simulink model "bh_2dof_NP_CONTROLLED"  (R2017a)
settings: Solver=ode45  StartTime=0.0  StopTime=70  FixedStep=0.001  RelTol=1e-7  EnableMultiTasking=on
values from neighbouring files (symbols this model uses):
  theta1_0 = 0    [bh_SIMPARAMS_for_2dof_NP_Control_sim.m]
  theta1_dot_0 = 0    [bh_SIMPARAMS_for_2dof_NP_Control_sim.m]
  theta4_0 = 0    [bh_SIMPARAMS_for_2dof_NP_Control_sim.m]
  theta4_dot_0 = 0    [bh_SIMPARAMS_for_2dof_NP_Control_sim.m]
undefined symbols (not defined in the file or in its folder): b1_damp, b4_damp, g, L1x, L1y, L1z, mass1, mass4, Rturn, sigbuilder_block
libraries: simulink_extras x18, simulink x4, discretizing x1
settings Model: Creator=bhorton  LastModifiedBy=bhorton
settings SolverCC: ZeroCrossAlgorithm=Adaptive
settings OptimizationCC: LifeSpan=inf
settings DebuggingCC: SFUnexpectedBacktrackingDiag=warning  SFNoUnconditionalDefaultTransitionDiag=warning  SFExecutionAtInitializationDiag=none
settings GRTTargetCC: TargetLangStandard=C89/C90 (ANSI)
settings ConfigComp: CovMetricSettings=dw  CovHtmlReporting=on  CovSaveCumulativeToWorkspaceVar=on  CovSaveSingleToWorkspaceVar=on  CovExternalEMLEnable=off
settings SimscapeCC: SimscapeLogDataHistory=10000  SelectedTab=Simscape Multibody
settings ExplorerConfigSet: InternalSimMechanicsExplorerSettings="<ExplorerConfiguration><canonicalview>default</canonicalview><AnimationSetting><BasePlaybackSpeed>2</BasePlaybackSpeed><PlaybackSpeedFactor>1.0</PlaybackSpeedFactor></AnimationSetting><TilePanel><TileInfo><Tiles Columns=\"1\" Count=\"1\" Rows=\"1\"><Column Left=\"2\" Weight=\"1\"/><Column Left=\"820\"/><Row Top=\"2\" Weight=\"1\"/><Row Top=\"545\"/><Tile Height=\"1\" Width=\"1\" X=\"0\" Y=\"0\"/></Tiles></TileInfo><SceneInfo><SceneViewer><BGColor><R>0.60000002384185791</R><G>0.60000002384185791</G><B>0.60000002384185791</B></BGColor><Camera><DoPerspective>off</DoPerspective><Position><X>0.3018347345439823</X><Y>0.024415264242792611</Y><Z>0.21433472519445274</Z></Position><Center><X>0.024999999062628675</X><Y>0.30124999972414623</Y><Z>-0.062500010286905439</Z></Center><Up><X>-0.40824829046386751</X><Y>0.40824829046386751</Y><Z>0.81649658092772159</Z></Up><ViewLimDist>1</ViewLimDist><YLim>0.27384785473346712</YLim><XLim>0.4148743716842227</XLim></Camera></SceneViewer></SceneInfo></TilePanel><MechEditorPanel><Cameras/><GfxPanelCameraMap/></MechEditorPanel></ExplorerConfiguration>"

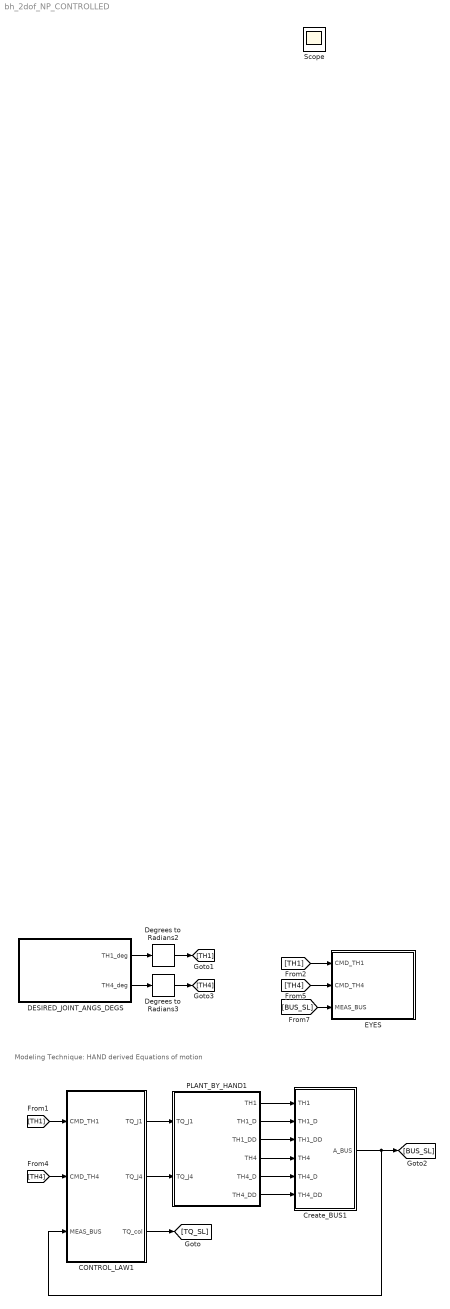
== system bh_2dof_NP_CONTROLLED ==
  note: Modeling Technique: HAND derived Equations of motion
  CONTROL_LAW1 : Subsystem
  Create_BUS1 : Subsystem
  DESIRED_JOINT_ANGS_DEGS : Subsystem  Tag=STV Subsys  LoadFcn=sigbuilder_block('load');  StartFcn=sigbuilder_block('start');  StopFcn=sigbuilder_block('stop');  ClipboardFcn=sigbuilder_block('clipboard');  mask(Sigbuilder block){tuvar=[0:10]}
      mask help: Simulink:masks:SigbuilderBlock_MD
      mask init:
      | if ~strcmp(get_param(bdroot(gcbh),'SimulationStatus'),'stopped') tuvar = sigbuilder_block('maskInit'); end
      settings: CopyFcn=sigbuilder_block('copy');  DeleteFcn=sigbuilder_block('delete');  ModelCloseFcn=sigbuilder_block('modelClose');  PreSaveFcn=sigbuilder_block('preSave');  PauseFcn=sigbuilder_block('pause');  ContinueFcn=sigbuilder_block('continue');  NameChangeFcn=sigbuilder_block('namechange');  OpenFcn=sigbuilder_block('open',[6 30 1428 681.75 ]);  CloseFcn=sigbuilder_block('close');
      mask Display: plot(0, 0, 100, 100,[2, 2, 32, 32, 2], [68, 8, 8, 68, 68],[32, 2], [38, 38], [32, 19, 2],[53, 60, 44], [32, 17, 17, 2],[16, 16, 31, 31]);txt = getActiveGroup(gcbh);text(2, 100, txt,'verticalAlignment', 'top');
  Degrees to Radians2 : simulink_extras/Transformations/Degrees to Radians
  Degrees to Radians3 : simulink_extras/Transformations/Degrees to Radians
  EYES : Subsystem
  PLANT_BY_HAND1 : Subsystem
  Scope : Scope
  wires:
  [TH1] -> EYES/1(CMD_TH1)
  [TH4] -> EYES/2(CMD_TH4)
  [TH1] -> CONTROL_LAW1/1(CMD_TH1)
  CONTROL_LAW1/3(TQ_col) -> [TQ_SL]
  PLANT_BY_HAND1/5(TH4_D) -> Create_BUS1/5(TH4_D)
  [TH4] -> CONTROL_LAW1/2(CMD_TH4)
  PLANT_BY_HAND1/3(TH1_DD) -> Create_BUS1/3(TH1_DD)
  PLANT_BY_HAND1/4(TH4) -> Create_BUS1/4(TH4)
  PLANT_BY_HAND1/1(TH1) -> Create_BUS1/1(TH1)
  PLANT_BY_HAND1/6(TH4_DD) -> Create_BUS1/6(TH4_DD)
  Create_BUS1/1(A_BUS) -> [BUS_SL], CONTROL_LAW1/3(MEAS_BUS)
  PLANT_BY_HAND1/2(TH1_D) -> Create_BUS1/2(TH1_D)
  CONTROL_LAW1/1(TQ_J1) -> PLANT_BY_HAND1/1("TQ_J1 ")
  CONTROL_LAW1/2(TQ_J4) -> PLANT_BY_HAND1/2(TQ_J4)
  [BUS_SL] -> EYES/3(MEAS_BUS)
  Degrees to Radians3/1 -> [TH4]
  DESIRED_JOINT_ANGS_DEGS/1(TH1_deg) -> Degrees to Radians2/1
  Degrees to Radians2/1 -> [TH1]
  DESIRED_JOINT_ANGS_DEGS/2(TH4_deg) -> Degrees to Radians3/1

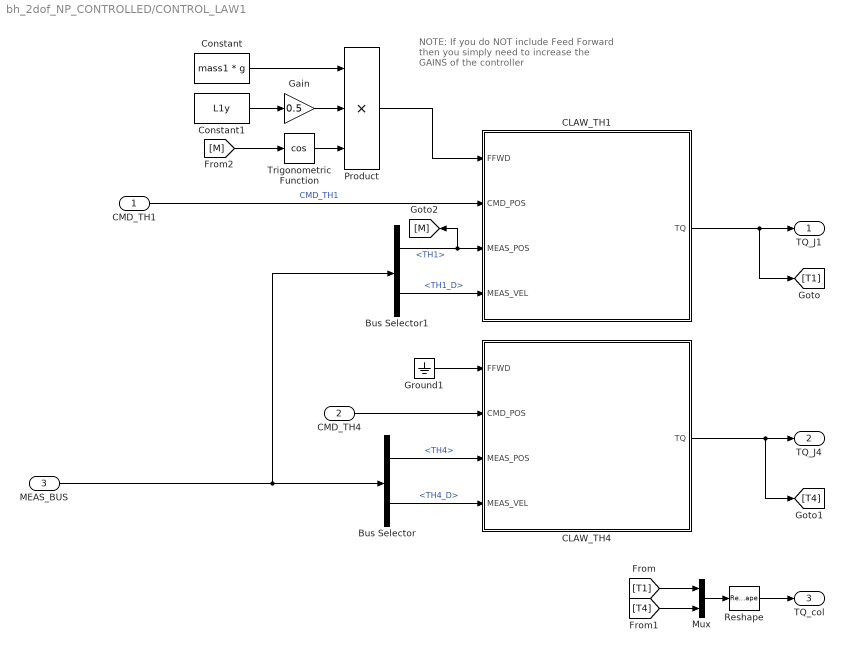
== system bh_2dof_NP_CONTROLLED/CONTROL_LAW1 ==
  note: NOTE:
      | If you do NOT include Feed Forward
      | then you simply need to increase the GAINS of the controller
  CMD_TH1 : Inport
  CMD_TH4 : Inport  Port=2
  MEAS_BUS : Inport  Port=3
  Bus Selector : BusSelector  OutputSignals=TH4,TH4_D
  Bus Selector1 : BusSelector  OutputSignals=TH1,TH1_D
  CLAW_TH1 : Subsystem
  CLAW_TH4 : Subsystem
  Constant : Constant  Value=mass1 * g
  Constant1 : Constant  Value=L1y
  Gain : Gain  Gain=0.5
  Ground1 : Ground
  Mux : Mux  Inputs=2
  Product : Product  Inputs=3
  Reshape : Reshape  OutputDimensionality=Column vector (2-D)
  Trigonometric Function : Trigonometry  Operator=cos
  TQ_J1 : Outport
  TQ_J4 : Outport  Port=2
  TQ_col : Outport  Port=3
  wires:
  MEAS_BUS/1 -> Bus Selector1/1, Bus Selector/1
  CMD_TH4/1 -> CLAW_TH4/2(CMD_POS)
  Bus Selector/2 -> CLAW_TH4/4(MEAS_VEL)  "<TH4_D>"
  Bus Selector/1 -> CLAW_TH4/3(MEAS_POS)  "<TH4>"
  Bus Selector1/1 -> [M], CLAW_TH1/3(MEAS_POS)  "<TH1>"
  Bus Selector1/2 -> CLAW_TH1/4(MEAS_VEL)  "<TH1_D>"
  CLAW_TH1/1(TQ) -> [T1], TQ_J1/1
  Ground1/1 -> CLAW_TH4/1(FFWD)
  CLAW_TH4/1(TQ) -> [T4], TQ_J4/1
  CMD_TH1/1 -> CLAW_TH1/2(CMD_POS)  "CMD_TH1"
  Constant/1 -> Product/1
  Constant1/1 -> Gain/1
  Product/1 -> CLAW_TH1/1(FFWD)
  Gain/1 -> Product/2
  Trigonometric Function/1 -> Product/3
  Mux/1 -> Reshape/1
  [T1] -> Mux/1
  [T4] -> Mux/2
  Reshape/1 -> TQ_col/1
  [M] -> Trigonometric Function/1

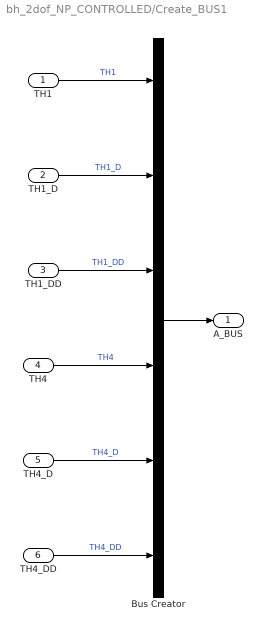
== system bh_2dof_NP_CONTROLLED/Create_BUS1 ==
  TH1 : Inport
  TH1_D : Inport  Port=2
  TH1_DD : Inport  Port=3
  TH4 : Inport  Port=4
  TH4_D : Inport  Port=5
  TH4_DD : Inport  Port=6
  Bus Creator : BusCreator  Inputs=6
  A_BUS : Outport
  wires:
  TH1_DD/1 -> Bus Creator/3  "TH1_DD"
  TH1_D/1 -> Bus Creator/2  "TH1_D"
  TH1/1 -> Bus Creator/1  "TH1"
  Bus Creator/1 -> A_BUS/1
  TH4_DD/1 -> Bus Creator/6  "TH4_DD"
  TH4_D/1 -> Bus Creator/5  "TH4_D"
  TH4/1 -> Bus Creator/4  "TH4"

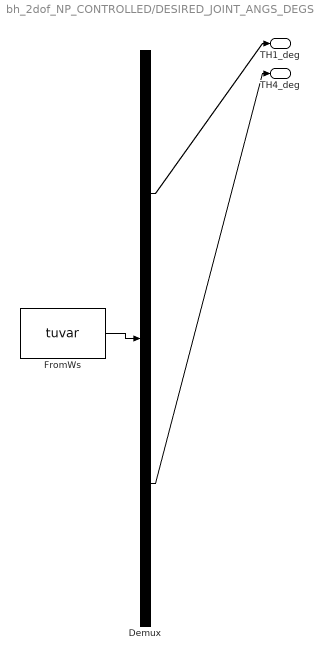
== system bh_2dof_NP_CONTROLLED/DESIRED_JOINT_ANGS_DEGS ==
  Demux : Demux  Tag=STV Demux  Outputs=2
  FromWs : FromWorkspace  Tag=STV FromWs  VariableName=tuvar  SampleTime=0
      SigBuilderData=|
      | common.afterFinalStr = 'Extrapolate'
      | common.sampleTime = 0
      | dataSet(1).timeRange = [0 60]
      | dataSet(1).name = 'SCENARIO_A_JUST_TH1'
      | dataSet(2).timeRange = [0 60]
      | dataSet(2).name = 'SCENARIO_B_JUST_TH4'
      | dataSet(3).timeRange = [0 60]
      | dataSet(3).name = 'SCENARIO_C_TH1_and_TH4'
      | dataSet(4).timeRange = [0 60]
      | dataSet(4).name = 'SCENARIO_D_TH1_and_TH4'
      | dataSet(5).timeRange = [0 70]
      | dataSet(5).name = 'SCENARIO_E'
      | sbobj.Groups(1).Name = 'SCENARIO_A_JUST_TH1'
      | sbobj.Groups(1).Signals(1).Name = 'TH1_deg'
      | sbobj.Groups(1).Signals(1).XData = [0 20 20 60]
      | sbobj.Groups(1).Signals(1).YData = [0 0 45 45]
      | sbobj.Groups(1).Signals(2).Name = 'TH4_deg'
      | sbobj.Groups(1).Signals(2).XData = [0 60]
      | sbobj.Groups(1).Signals(2).YData = [0 0]
      | sbobj.Groups(1).TimeRange = [0 60]
      | sbobj.Groups(2).Name = 'SCENARIO_B_JUST_TH4'
      | sbobj.Groups(2).Signals(1).Name = 'TH1_deg'
      | sbobj.Groups(2).Signals(1).XData = [0 20 60]
      | sbobj.Groups(2).Signals(1).YData = [0 0 0]
      | sbobj.Groups(2).Signals(2).Name = 'TH4_deg'
      | sbobj.Groups(2).Signals(2).XData = [0 20 20 60]
      | sbobj.Groups(2).Signals(2).YData = [0 0 45 45]
      | sbobj.Groups(2).TimeRange = [0 60]
      | sbobj.Groups(3).Name = 'SCENARIO_C_TH1_and_TH4'
      | sbobj.Groups(3).Signals(1).Name = 'TH1_deg'
      | sbobj.Groups(3).Signals(1).XData = [0 10 10 40 60]
      | sbobj.Groups(3).Signals(1).YData = [0 0 45 45 0]
      | sbobj.Groups(3).Signals(2).Name = 'TH4_deg'
      | sbobj.Groups(3).Signals(2).XData = [0 14.95 14.95 30 60]
      | sbobj.Groups(3).Signals(2).YData = [0 0 45 45 0]
      | sbobj.Groups(3).TimeRange = [0 60]
      | sbobj.Groups(4).Name = 'SCENARIO_D_TH1_and_TH4'
      | sbobj.Groups(4).Signals(1).Name = 'TH1_deg'
      | sbobj.Groups(4).Signals(1).XData = [0 10 40 60]
      | sbobj.Groups(4).Signals(1).YData = [0 45 45 0]
      | sbobj.Groups(4).Signals(2).Name = 'TH4_deg'
      | sbobj.Groups(4).Signals(2).XData = [0 10 30 60]
      | sbobj.Groups(4).Signals(2).YData = [0 45 45 0]
      | sbobj.Groups(4).TimeRange = [0 60]
      | sbobj.Groups(5).Name = 'SCENARIO_E'
      | sbobj.Groups(5).Signals(1).Name = 'TH1_deg'
      | sbobj.Groups(5).Signals(1).XData = [0 35.15 45.4 60 70]
      | sbobj.Groups(5).Signals(1).YData = [0 0 45 -45 0]
      | sbobj.Groups(5).Signals(2).Name = 'TH4_deg'
      | sbobj.Groups(5).Signals(2).XData = [0 10 25 30 70]
      | sbobj.Groups(5).Signals(2).YData = [0 -90 90 0 0]
      | sbobj.Groups(5).TimeRange = [0 70]
  TH1_deg : Outport  Tag=STV Outport
  TH4_deg : Outport  Tag=STV Outport  Port=2
  wires:
  FromWs/1 -> Demux/1
  Demux/1 -> TH1_deg/1
  Demux/2 -> TH4_deg/1

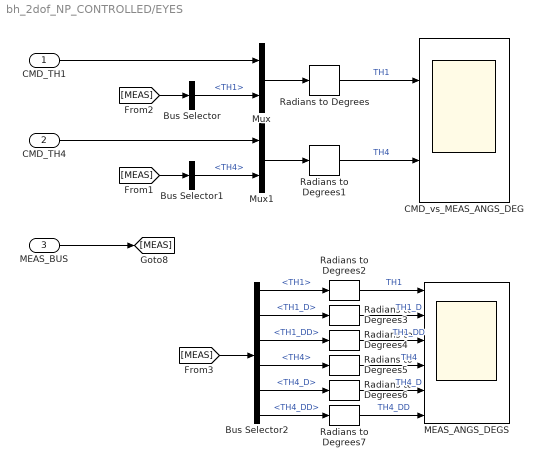
== system bh_2dof_NP_CONTROLLED/EYES ==
  CMD_TH1 : Inport
  CMD_TH4 : Inport  Port=2
  MEAS_BUS : Inport  Port=3
  Bus Selector : BusSelector  OutputSignals=TH1
  Bus Selector1 : BusSelector  OutputSignals=TH4
  Bus Selector2 : BusSelector  OutputSignals=TH1,TH1_D,TH1_DD,TH4,TH4_D,TH4_DD
  CMD_vs_MEAS_ANGS_DEG : Scope  NumInputPorts=2
  MEAS_ANGS_DEGS : Scope  NumInputPorts=6
  Mux : Mux  Inputs=2
  Mux1 : Mux  Inputs=2
  Radians to Degrees{,1..7} (8 alike) : simulink_extras/Transformations/Radians to Degrees
  wires:
  MEAS_BUS/1 -> [MEAS]
  CMD_TH1/1 -> Mux/1
  Bus Selector/1 -> Mux/2  "<TH1>"
  [MEAS] -> Bus Selector/1
  Mux/1 -> Radians to Degrees/1
  CMD_TH4/1 -> Mux1/1
  Bus Selector1/1 -> Mux1/2  "<TH4>"
  [MEAS] -> Bus Selector1/1
  Mux1/1 -> Radians to Degrees1/1
  Radians to Degrees1/1 -> CMD_vs_MEAS_ANGS_DEG/2  "TH4"
  Radians to Degrees/1 -> CMD_vs_MEAS_ANGS_DEG/1  "TH1"
  [MEAS] -> Bus Selector2/1
  Bus Selector2/6 -> Radians to Degrees7/1  "<TH4_DD>"
  Bus Selector2/3 -> Radians to Degrees4/1  "<TH1_DD>"
  Bus Selector2/4 -> Radians to Degrees5/1  "<TH4>"
  Bus Selector2/5 -> Radians to Degrees6/1  "<TH4_D>"
  Bus Selector2/2 -> Radians to Degrees3/1  "<TH1_D>"
  Bus Selector2/1 -> Radians to Degrees2/1  "<TH1>"
  Radians to Degrees2/1 -> MEAS_ANGS_DEGS/1  "TH1"
  Radians to Degrees3/1 -> MEAS_ANGS_DEGS/2  "TH1_D"
  Radians to Degrees4/1 -> MEAS_ANGS_DEGS/3  "TH1_DD"
  Radians to Degrees5/1 -> MEAS_ANGS_DEGS/4  "TH4"
  Radians to Degrees6/1 -> MEAS_ANGS_DEGS/5  "TH4_D"
  Radians to Degrees7/1 -> MEAS_ANGS_DEGS/6  "TH4_DD"

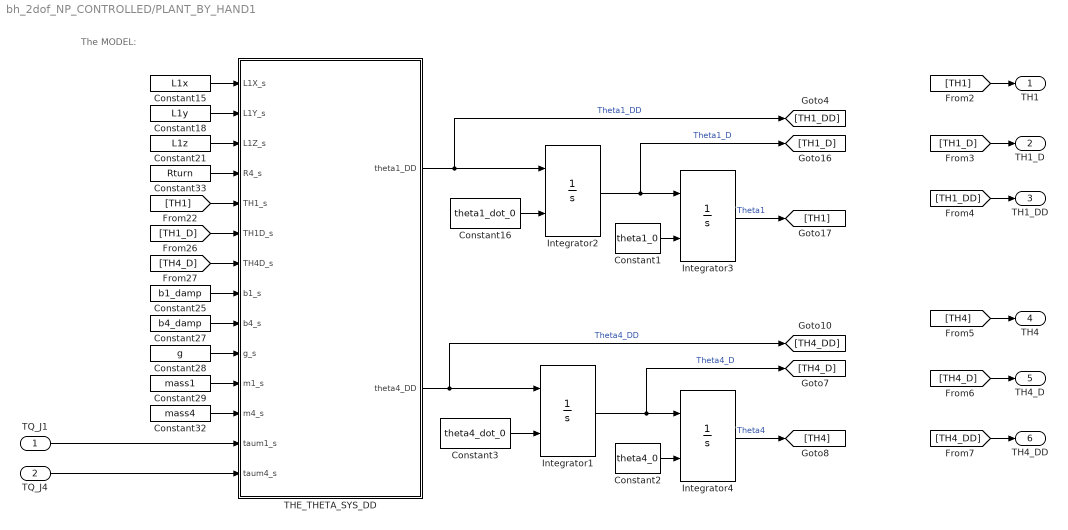
== system bh_2dof_NP_CONTROLLED/PLANT_BY_HAND1 ==
  note: The MODEL:
  "TQ_J1 " : Inport
  TQ_J4 : Inport  Port=2
  Constant1 : Constant  Value=theta1_0
  Constant15 : Constant  Value=L1x
  Constant16 : Constant  Value=theta1_dot_0
  Constant18 : Constant  Value=L1y
  Constant2 : Constant  Value=theta4_0
  Constant21 : Constant  Value=L1z
  Constant25 : Constant  Value=b1_damp
  Constant27 : Constant  Value=b4_damp
  Constant28 : Constant  Value=g
  Constant29 : Constant  Value=mass1
  Constant3 : Constant  Value=theta4_dot_0
  Constant32 : Constant  Value=mass4
  Constant33 : Constant  Value=Rturn
  Integrator{1..4} (4 alike) : Integrator  InitialConditionSource=external
  THE_THETA_SYS_DD : MATLAB Function  TreatAsAtomicUnit=on
  TH1 : Outport
  TH1_D : Outport  Port=2
  TH1_DD : Outport  Port=3
  TH4 : Outport  Port=4
  TH4_D : Outport  Port=5
  TH4_DD : Outport  Port=6
  wires:
  [TH4_D] -> TH4_D/1
  Constant16/1 -> Integrator2/2
  Integrator2/1 -> [TH1_D], Integrator3/1  "Theta1_D"
  TQ_J4/1 -> THE_THETA_SYS_DD/14(taum4_s)
  Integrator4/1 -> [TH4]  "Theta4"
  [TH4_D] -> THE_THETA_SYS_DD/7(TH4D_s)
  [TH1] -> THE_THETA_SYS_DD/5(TH1_s)
  [TH1_DD] -> TH1_DD/1
  Constant29/1 -> THE_THETA_SYS_DD/11(m1_s)
  Constant33/1 -> THE_THETA_SYS_DD/4(R4_s)
  THE_THETA_SYS_DD/1(theta1_DD) -> [TH1_DD], Integrator2/1  "Theta1_DD"
  Integrator3/1 -> [TH1]  "Theta1"
  Constant18/1 -> THE_THETA_SYS_DD/2(L1Y_s)
  THE_THETA_SYS_DD/2(theta4_DD) -> Integrator1/1, [TH4_DD]  "Theta4_DD"
  Constant2/1 -> Integrator4/2
  "TQ_J1 "/1 -> THE_THETA_SYS_DD/13(taum1_s)
  [TH1] -> TH1/1
  Constant1/1 -> Integrator3/2
  Constant27/1 -> THE_THETA_SYS_DD/9(b4_s)
  [TH1_D] -> TH1_D/1
  Constant32/1 -> THE_THETA_SYS_DD/12(m4_s)
  [TH4_DD] -> TH4_DD/1
  Constant3/1 -> Integrator1/2
  Constant25/1 -> THE_THETA_SYS_DD/8(b1_s)
  [TH4] -> TH4/1
  Constant15/1 -> THE_THETA_SYS_DD/1(L1X_s)
  Constant21/1 -> THE_THETA_SYS_DD/3(L1Z_s)
  [TH1_D] -> THE_THETA_SYS_DD/6(TH1D_s)
  Integrator1/1 -> [TH4_D], Integrator4/1  "Theta4_D"
  Constant28/1 -> THE_THETA_SYS_DD/10(g_s)

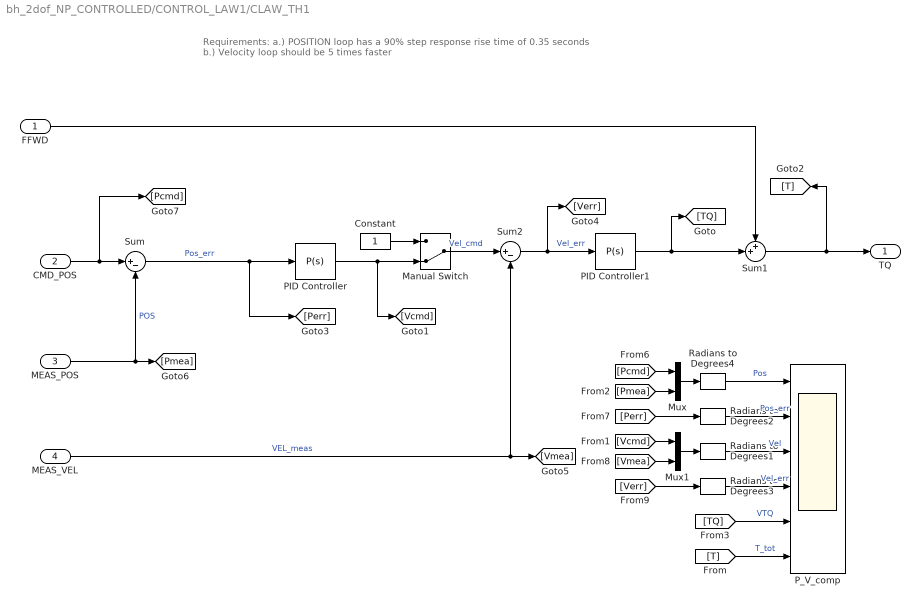
== system bh_2dof_NP_CONTROLLED/CONTROL_LAW1/CLAW_TH1 ==
  note: Requirements:
      | a.) POSITION loop has a 90% step response
      | rise time of 0.35 seconds
      |
      | b.) Velocity loop should be 5 times faster
  FFWD : Inport
  CMD_POS : Inport  Port=2
  MEAS_POS : Inport  Port=3
  MEAS_VEL : Inport  Port=4
  Constant : Constant
  Manual Switch : ManualSwitch  CurrentSetting=0
  Mux : Mux  Inputs=2
  Mux1 : Mux  Inputs=2
  PID Controller : simulink/Continuous/PID Controller  Controller=P  TimeDomain=Continuous-time  SampleTime=-1  IntegratorMethod=Forward Euler  FilterMethod=Forward Euler  Form=Parallel  UseFilter=on  ControllerParametersSource=internal  P=5.58549433794614  I=0  D=0  N=100  InitialConditionSource=internal  InitialConditionForIntegrator=0  InitialConditionForFilter=0  ExternalReset=none  LimitOutput=off  UpperSaturationLimit=inf  LowerSaturationLimit=-inf  LinearizeAsGain=on  AntiWindupMode=none  Kb=1  TrackingMode=off  Kt=1  PParamMin=[]  PParamMax=[]  IParamMin=[]  IParamMax=[]  DParamMin=[]  DParamMax=[]  NParamMin=[]  NParamMax=[]  KbParamMin=[]  KbParamMax=[]  KtParamMin=[]  KtParamMax=[]  POutMin=[]  POutMax=[]  IOutMin=[]  IOutMax=[]  DOutMin=[]  DOutMax=[]  NOutMin=[]  NOutMax=[]  KbOutMin=[]  KbOutMax=[]  KtOutMin=[]  KtOutMax=[]  IntegratorOutMin=[]  IntegratorOutMax=[]  FilterOutMin=[]  FilterOutMax=[]  SumOutMin=[]  SumOutMax=[]  SumI1OutMin=[]  SumI1OutMax=[]  SumI2OutMin=[]  SumI2OutMax=[]  SumI3OutMin=[]  SumI3OutMax=[]  SumDOutMin=[]  SumDOutMax=[]  SaturationOutMin=[]  SaturationOutMax=[]  IntegratorContinuousStateAttributes=''  IntegratorStateMustResolveToSignalObject=off  IntegratorRTWStateStorageClass=Auto  FilterContinuousStateAttributes=''  FilterStateMustResolveToSignalObject=off  FilterRTWStateStorageClass=Auto  DifferentiatorICPrevScaledInput=0  DifferentiatorOutMin=[]  DifferentiatorOutMax=[]  InitialConditionSetting=State (most efficient)
  PID Controller1 : simulink/Continuous/PID Controller  Controller=P  TimeDomain=Continuous-time  SampleTime=-1  IntegratorMethod=Forward Euler  FilterMethod=Forward Euler  Form=Parallel  UseFilter=on  ControllerParametersSource=internal  P=1  I=1  D=0  N=100  InitialConditionSource=internal  InitialConditionForIntegrator=0  InitialConditionForFilter=0  ExternalReset=none  LimitOutput=off  UpperSaturationLimit=inf  LowerSaturationLimit=-inf  LinearizeAsGain=on  AntiWindupMode=none  Kb=1  TrackingMode=off  Kt=1  PParamMin=[]  PParamMax=[]  IParamMin=[]  IParamMax=[]  DParamMin=[]  DParamMax=[]  NParamMin=[]  NParamMax=[]  KbParamMin=[]  KbParamMax=[]  KtParamMin=[]  KtParamMax=[]  POutMin=[]  POutMax=[]  IOutMin=[]  IOutMax=[]  DOutMin=[]  DOutMax=[]  NOutMin=[]  NOutMax=[]  KbOutMin=[]  KbOutMax=[]  KtOutMin=[]  KtOutMax=[]  IntegratorOutMin=[]  IntegratorOutMax=[]  FilterOutMin=[]  FilterOutMax=[]  SumOutMin=[]  SumOutMax=[]  SumI1OutMin=[]  SumI1OutMax=[]  SumI2OutMin=[]  SumI2OutMax=[]  SumI3OutMin=[]  SumI3OutMax=[]  SumDOutMin=[]  SumDOutMax=[]  SaturationOutMin=[]  SaturationOutMax=[]  IntegratorContinuousStateAttributes=''  IntegratorStateMustResolveToSignalObject=off  IntegratorRTWStateStorageClass=Auto  FilterContinuousStateAttributes=''  FilterStateMustResolveToSignalObject=off  FilterRTWStateStorageClass=Auto  DifferentiatorICPrevScaledInput=0  DifferentiatorOutMin=[]  DifferentiatorOutMax=[]  InitialConditionSetting=State (most efficient)
  P_V_comp : Scope  NumInputPorts=6
  Radians to Degrees{1..4} (4 alike) : simulink_extras/Transformations/Radians to Degrees
  Sum : Sum  Inputs=|+-
  Sum1 : Sum  Inputs=++|
  Sum2 : Sum  Inputs=|+-
  TQ : Outport
  wires:
  FFWD/1 -> Sum1/1
  CMD_POS/1 -> [Pcmd], Sum/1
  MEAS_VEL/1 -> [Vmea], Sum2/2  "VEL_meas"
  MEAS_POS/1 -> [Pmea], Sum/2  "POS"
  Sum2/1 -> PID Controller1/1, [Verr]  "Vel_err"
  Manual Switch/1 -> Sum2/1  "Vel_cmd"
  Constant/1 -> Manual Switch/1
  Sum/1 -> PID Controller/1, [Perr]  "Pos_err"
  PID Controller/1 -> Manual Switch/2, [Vcmd]
  Sum1/1 -> TQ/1, [T]
  Mux/1 -> Radians to Degrees4/1
  [Pcmd] -> Mux/1
  [Pmea] -> Mux/2
  Mux1/1 -> Radians to Degrees1/1
  [Vcmd] -> Mux1/1
  [Vmea] -> Mux1/2
  [Verr] -> Radians to Degrees3/1
  [Perr] -> Radians to Degrees2/1
  Radians to Degrees3/1 -> P_V_comp/4  "Vel_err"
  Radians to Degrees2/1 -> P_V_comp/2  "Pos_err"
  Radians to Degrees1/1 -> P_V_comp/3  "Vel"
  Radians to Degrees4/1 -> P_V_comp/1  "Pos"
  [TQ] -> P_V_comp/5  "VTQ"
  [T] -> P_V_comp/6  "T_tot"
  PID Controller1/1 -> Sum1/2, [TQ]

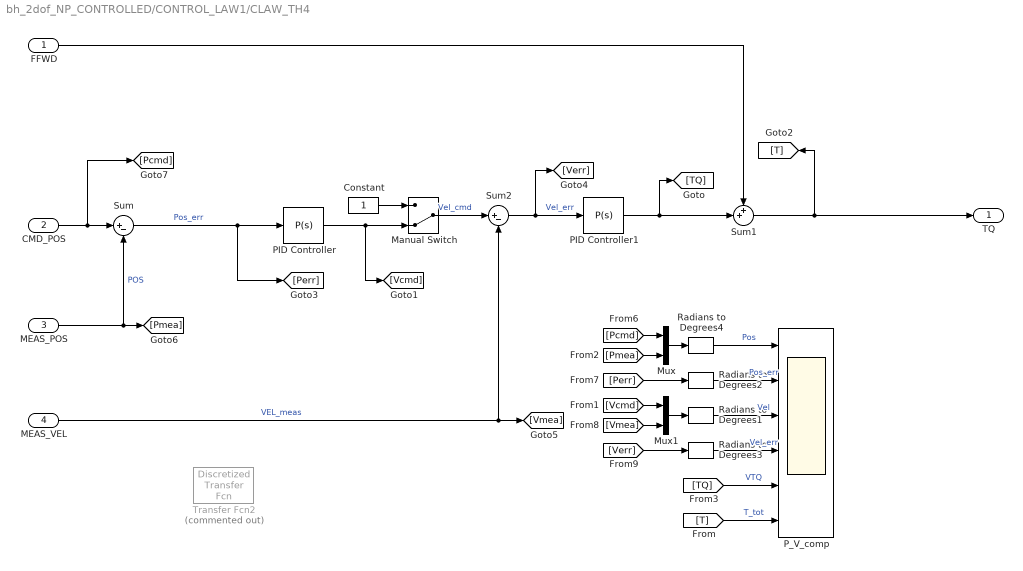
== system bh_2dof_NP_CONTROLLED/CONTROL_LAW1/CLAW_TH4 ==
  FFWD : Inport
  CMD_POS : Inport  Port=2
  MEAS_POS : Inport  Port=3
  MEAS_VEL : Inport  Port=4
  Constant : Constant
  Manual Switch : ManualSwitch  CurrentSetting=0
  Mux : Mux  Inputs=2
  Mux1 : Mux  Inputs=2
  PID Controller : simulink/Continuous/PID Controller  Controller=P  TimeDomain=Continuous-time  SampleTime=-1  IntegratorMethod=Forward Euler  FilterMethod=Forward Euler  Form=Parallel  UseFilter=on  ControllerParametersSource=internal  P=5.58549433794614  I=1  D=0  N=100  InitialConditionSource=internal  InitialConditionForIntegrator=0  InitialConditionForFilter=0  ExternalReset=none  LimitOutput=off  UpperSaturationLimit=inf  LowerSaturationLimit=-inf  LinearizeAsGain=on  AntiWindupMode=none  Kb=1  TrackingMode=off  Kt=1  PParamMin=[]  PParamMax=[]  IParamMin=[]  IParamMax=[]  DParamMin=[]  DParamMax=[]  NParamMin=[]  NParamMax=[]  KbParamMin=[]  KbParamMax=[]  KtParamMin=[]  KtParamMax=[]  POutMin=[]  POutMax=[]  IOutMin=[]  IOutMax=[]  DOutMin=[]  DOutMax=[]  NOutMin=[]  NOutMax=[]  KbOutMin=[]  KbOutMax=[]  KtOutMin=[]  KtOutMax=[]  IntegratorOutMin=[]  IntegratorOutMax=[]  FilterOutMin=[]  FilterOutMax=[]  SumOutMin=[]  SumOutMax=[]  SumI1OutMin=[]  SumI1OutMax=[]  SumI2OutMin=[]  SumI2OutMax=[]  SumI3OutMin=[]  SumI3OutMax=[]  SumDOutMin=[]  SumDOutMax=[]  SaturationOutMin=[]  SaturationOutMax=[]  IntegratorContinuousStateAttributes=''  IntegratorStateMustResolveToSignalObject=off  IntegratorRTWStateStorageClass=Auto  FilterContinuousStateAttributes=''  FilterStateMustResolveToSignalObject=off  FilterRTWStateStorageClass=Auto  DifferentiatorICPrevScaledInput=0  DifferentiatorOutMin=[]  DifferentiatorOutMax=[]  InitialConditionSetting=State (most efficient)
  PID Controller1 : simulink/Continuous/PID Controller  Controller=P  TimeDomain=Continuous-time  SampleTime=-1  IntegratorMethod=Forward Euler  FilterMethod=Forward Euler  Form=Parallel  UseFilter=on  ControllerParametersSource=internal  P=1  I=1  D=0  N=100  InitialConditionSource=internal  InitialConditionForIntegrator=0  InitialConditionForFilter=0  ExternalReset=none  LimitOutput=off  UpperSaturationLimit=inf  LowerSaturationLimit=-inf  LinearizeAsGain=on  AntiWindupMode=none  Kb=1  TrackingMode=off  Kt=1  PParamMin=[]  PParamMax=[]  IParamMin=[]  IParamMax=[]  DParamMin=[]  DParamMax=[]  NParamMin=[]  NParamMax=[]  KbParamMin=[]  KbParamMax=[]  KtParamMin=[]  KtParamMax=[]  POutMin=[]  POutMax=[]  IOutMin=[]  IOutMax=[]  DOutMin=[]  DOutMax=[]  NOutMin=[]  NOutMax=[]  KbOutMin=[]  KbOutMax=[]  KtOutMin=[]  KtOutMax=[]  IntegratorOutMin=[]  IntegratorOutMax=[]  FilterOutMin=[]  FilterOutMax=[]  SumOutMin=[]  SumOutMax=[]  SumI1OutMin=[]  SumI1OutMax=[]  SumI2OutMin=[]  SumI2OutMax=[]  SumI3OutMin=[]  SumI3OutMax=[]  SumDOutMin=[]  SumDOutMax=[]  SaturationOutMin=[]  SaturationOutMax=[]  IntegratorContinuousStateAttributes=''  IntegratorStateMustResolveToSignalObject=off  IntegratorRTWStateStorageClass=Auto  FilterContinuousStateAttributes=''  FilterStateMustResolveToSignalObject=off  FilterRTWStateStorageClass=Auto  DifferentiatorICPrevScaledInput=0  DifferentiatorOutMin=[]  DifferentiatorOutMax=[]  InitialConditionSetting=State (most efficient)
  P_V_comp : Scope  NumInputPorts=6
  Radians to Degrees{1..4} (4 alike) : simulink_extras/Transformations/Radians to Degrees
  Sum : Sum  Inputs=|+-
  Sum1 : Sum  Inputs=++|
  Sum2 : Sum  Inputs=|+-
  Transfer Fcn2 : discretizing/Discretized Transfer Fcn  Commented=on  Numerator=[100]  Denominator=[1 100]  AbsTol=auto  SampleTime=0.001  method=tustin  Wc=1
  TQ : Outport
  wires:
  FFWD/1 -> Sum1/1
  CMD_POS/1 -> [Pcmd], Sum/1
  MEAS_VEL/1 -> [Vmea], Sum2/2  "VEL_meas"
  MEAS_POS/1 -> [Pmea], Sum/2  "POS"
  Sum2/1 -> PID Controller1/1, [Verr]  "Vel_err"
  Manual Switch/1 -> Sum2/1  "Vel_cmd"
  Constant/1 -> Manual Switch/1
  Sum/1 -> PID Controller/1, [Perr]  "Pos_err"
  PID Controller/1 -> Manual Switch/2, [Vcmd]
  Sum1/1 -> TQ/1, [T]
  Mux/1 -> Radians to Degrees4/1
  [Pcmd] -> Mux/1
  [Pmea] -> Mux/2
  Mux1/1 -> Radians to Degrees1/1
  [Vcmd] -> Mux1/1
  [Vmea] -> Mux1/2
  [Verr] -> Radians to Degrees3/1
  [Perr] -> Radians to Degrees2/1
  Radians to Degrees3/1 -> P_V_comp/4  "Vel_err"
  Radians to Degrees2/1 -> P_V_comp/2  "Pos_err"
  Radians to Degrees1/1 -> P_V_comp/3  "Vel"
  Radians to Degrees4/1 -> P_V_comp/1  "Pos"
  [TQ] -> P_V_comp/5  "VTQ"
  [T] -> P_V_comp/6  "T_tot"
  PID Controller1/1 -> Sum1/2, [TQ]

== matlab function bh_2dof_NP_CONTROLLED/PLANT_BY_HAND1/THE_THETA_SYS_DD ==
  data: L1X_s input; theta1_DD output; L1Y_s input; L1Z_s input; R4_s input; TH1_s input; TH1D_s input; TH4D_s input; b1_s input; b4_s input; g_s input; m1_s input; m4_s input; taum1_s input; taum4_s input; theta4_DD output
function [theta1_DD,theta4_DD] = THE_THETA_SYS_DD(L1X_s,L1Y_s,L1Z_s,R4_s,TH1_s,TH1D_s,TH4D_s,b1_s,b4_s,g_s,m1_s,m4_s,taum1_s,taum4_s)
%#codegen

%    This function was generated by the Symbolic Math Toolbox version 7.2.
%    19-Jul-2017 16:42:27

theta1_DD = (taum1_s.*1.2e1-TH1D_s.*b1_s.*1.2e1-L1Y_s.*g_s.*m1_s.*cos(TH1_s).*6.0-L1Y_s.^2.*TH4D_s.^2.*m1_s.*sin(TH1_s.*2.0).*2.0+L1Z_s.^2.*TH4D_s.^2.*m1_s.*sin(TH1_s.*2.0).*(1.0./2.0))./(L1Y_s.^2.*m1_s.*4.0+L1Z_s.^2.*m1_s);
if nargout > 1
    theta4_DD = (taum4_s.*2.4e1-TH4D_s.*b4_s.*2.4e1+L1Y_s.^2.*TH1D_s.*TH4D_s.*m1_s.*sin(TH1_s.*2.0).*8.0-L1Z_s.^2.*TH1D_s.*TH4D_s.*m1_s.*sin(TH1_s.*2.0).*2.0)./(L1X_s.^2.*m1_s.*2.0+L1Y_s.^2.*m1_s.*4.0+L1Z_s.^2.*m1_s+R4_s.^2.*m4_s.*1.2e1+L1Y_s.^2.*m1_s.*cos(TH1_s.*2.0).*4.0-L1Z_s.^2.*m1_s.*cos(TH1_s.*2.0));
end
